simulink model "accurateManipulatorModel"  (R2020b)
settings: Solver=VariableStepAuto  StartTime=0.0  StopTime=10.0  RelTol=1e-3
PreLoadFcn:
  | initModelData
values from neighbouring files (symbols this model uses):
  Bm = 4e-4    (= 0.0004)    [initModelData.m]
  Jm = 6.1e-4    (= 0.00061)    [initModelData.m]
  Kb = 0.105    [initModelData.m]
  Km = 0.105    [initModelData.m]
  L = 0.9e-3    (= 0.0009)    [initModelData.m]
  R = 0.76    [initModelData.m]
settings Model: Creator=esdan  LastModifiedBy=esdan

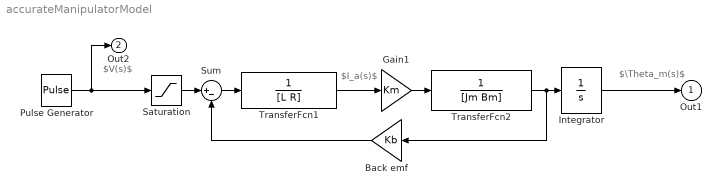
== system accurateManipulatorModel ==
  note: $I_a(s)$
  note: $\Theta_m(s)$
  note: $V(s)$
  Back emf : Gain  Gain=Kb
  Gain1 : Gain  Gain=Km
  Integrator : Integrator
  Pulse Generator : DiscretePulseGenerator  PulseType=Time based  Period=10  PulseWidth=33
  Saturation : Saturate  UpperLimit=35  LowerLimit=-35
  Sum : Sum  Inputs=|+-
  TransferFcn1 : TransferFcn  Denominator=[L R]
  TransferFcn2 : TransferFcn  Denominator=[Jm Bm]
  Out1 : Outport  SignalName=posAccurate
  Out2 : Outport  Port=2  SignalName=V
  wires:
  TransferFcn1/1 -> Gain1/1
  Pulse Generator/1 -> Saturation/1, Out2/1
  Sum/1 -> TransferFcn1/1
  TransferFcn2/1 -> Back emf/1, Integrator/1
  Gain1/1 -> TransferFcn2/1
  Integrator/1 -> Out1/1
  Back emf/1 -> Sum/2
  Saturation/1 -> Sum/1
